simulink model "sampleModel223"  (R2021b)
settings: Solver=VariableStepAuto  StartTime=0.0  StopTime=10.0  RelTol=1e-3
undefined symbols (not defined in the file or in its folder): DiscIntNeverNeededParam
libraries: simulink x6
settings Model: Creator=user  LastModifiedBy=user

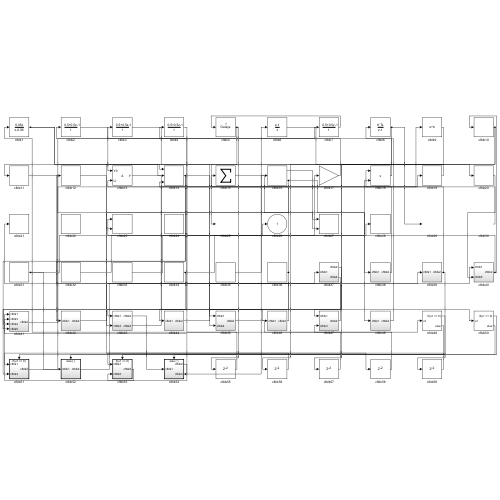
[thumbnail: Simulink's stored preview of the top-level diagram]
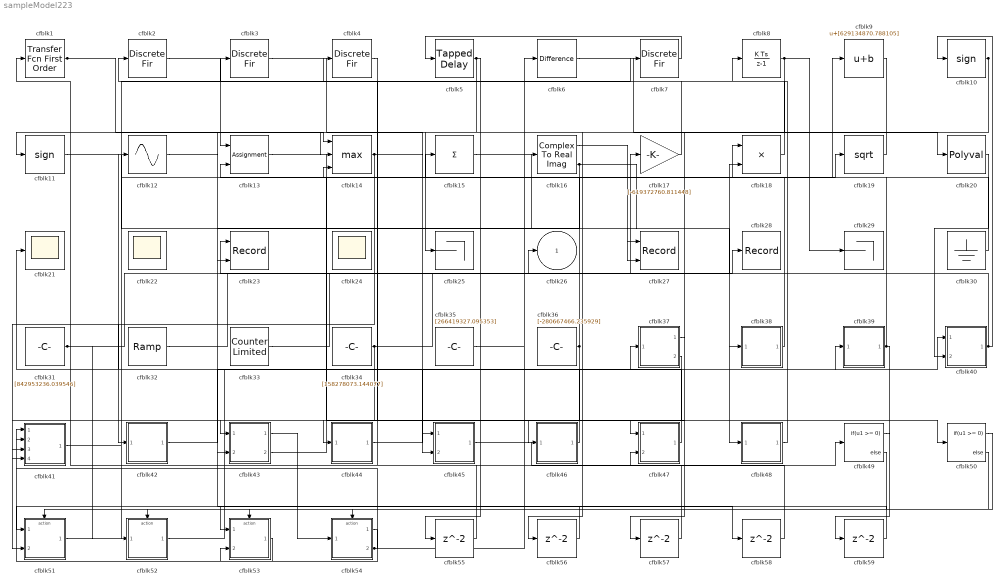
== system sampleModel223 ==
  cfblk1 : simulink/Discrete/Transfer Fcn First Order  PoleZ=0.95  ICPrevOutput=0.0  DoSatur=off
  cfblk10 : Signum
  cfblk11 : Signum
  cfblk12 : Sin  TimeSource=Use external signal  SampleTime=0
  cfblk13 : Assignment  DiagnosticForDimensions=Warning  IndexOptions=Index vector (dialog)  Indices=1  OutputSizes=1
  cfblk14 : MinMax  Function=max  Inputs=3
  cfblk15 : Sum  Inputs=+
  cfblk16 : ComplexToRealImag
  cfblk17 : Gain  Gain=[-619372760.811448]
  cfblk18 : Product
  cfblk19 : Sqrt  SaturateOnIntegerOverflow=on
  cfblk{2..4,7} (4 alike) : DiscreteFir  SampleTime=1
  cfblk20 : Polyval  Coefs=[ +2.081618890e-019, -1.441693666e-014, +4.719686976e-010, -8.536869453e-006, +1.621573104e-001, -8.087801117e+001 ]
  cfblk21 : Scope
  cfblk22 : Scope
      settings: Floating=on
  cfblk23 : Record  FileSettingsInternal="{\"entries\":[{\"content\":{\"excelSettings\":{\"content\":{},\"type\":\"Streamout.ExcelSettings\"}},\"type\":\"Streamout.FileSettingStorage\",\"uuid\":\"0ee5e5d3-5951-4c48-9d89-32d8b12ba518\"}],\"packageUris\":[\"http://schema.mathworks.com/mf0/streamout_blocks/R2020a\"],\"version\":\"1.0\"}"  Layout=[1 1]  SignalsInternal="{\"entries\":[{\"content\":{\"signals\":[{\"content\":{\"blockPath\":[\"sampleModel223/cfblk23\"],\"channel\":[],\"dimensions\":[1],\"domain\":\"sampleModel223/cfblk23\",\"lineColor\":\"#a2142f\",\"plots\":[1],\"port\":1,\"sid\":[\"\"],\"signalID\":8702,\"signalName\":\"cfblk40\"},\"type\":\"RecordBlkView.Signal\",\"uuid\":\"30bc6bd1-39a8-4b59-9cbd-2b18e3afbf50\"},{\"content\":{\"blockPath\":[\"sampleModel223/cfblk23\"],\"channel\":[],\"dimensions\":[1],\"domain\":\"sampleModel223/cfblk23\",\"lineColor\":\"#139fff\",\"plots\":[1],\"port\":2,\"sid\":[\"\"],\"signalID\":8706,\"signalName\":\"cfblk16:2\"},\"type\":\"RecordBlkView.Signal\",\"uuid\":\"da769030-c28c-44c7-86a2-4d1f259b478e\"}]},\"type\":\"RecordBlkView.InputSignals\",\"uuid\":\"dad23ff0-d1d3-46bd-a827-64e16703a200\"}],\"packageUris\":[\"http://schema.mathworks.com/mf0/streamout_blocks/R2020a\"],\"version\":\"1.0\"}"  VisualizationBindings="{\"xyplotplugin\":{\"info\":[{\"series\":[{\"bindingParametersList\":[{\"parameter\":\"X-Axis\",\"signalID\":8702,\"signalName\":\"cfblk40\"},{\"parameter\":\"Y-Axis\",\"signalID\":8706,\"signalName\":\"cfblk16:2\"}],\"seriesID\":59310}],\"subplotID\":1}]}}"  CompatibilityTag=XY
  cfblk24 : Scope
      settings: Floating=on
  cfblk25 : Terminator
  cfblk27 : Record  FileSettingsInternal="{\"entries\":[{\"content\":{\"excelSettings\":{\"content\":{},\"type\":\"Streamout.ExcelSettings\"}},\"type\":\"Streamout.FileSettingStorage\",\"uuid\":\"b9045ad8-1652-4b93-96d3-11a4ff897f15\"}],\"packageUris\":[\"http://schema.mathworks.com/mf0/streamout_blocks/R2020a\"],\"version\":\"1.0\"}"  Layout=[1 1]  SignalsInternal="{\"entries\":[{\"content\":{\"signals\":[{\"content\":{\"blockPath\":[\"sampleModel223/cfblk27\"],\"channel\":[],\"dimensions\":[1],\"domain\":\"sampleModel223/cfblk27\",\"lineColor\":\"#a2142f\",\"plots\":[1],\"port\":1,\"sid\":[\"\"],\"signalID\":8710,\"signalName\":\"cfblk16:1\"},\"type\":\"RecordBlkView.Signal\",\"uuid\":\"1ed41653-2a62-4b63-b81e-2f1a57827a1a\"},{\"content\":{\"blockPath\":[\"sampleModel223/cfblk27\"],\"channel\":[],\"dimensions\":[1],\"domain\":\"sampleModel223/cfblk27\",\"lineColor\":\"#139fff\",\"plots\":[1],\"port\":2,\"sid\":[\"\"],\"signalID\":8714,\"signalName\":\"cfblk11\"},\"type\":\"RecordBlkView.Signal\",\"uuid\":\"408a8370-a751-4b9d-9405-1cbd384d5eae\"}]},\"type\":\"RecordBlkView.InputSignals\",\"uuid\":\"9255ecad-2c20-41ba-b360-5dd1c328ef31\"}],\"packageUris\":[\"http://schema.mathworks.com/mf0/streamout_blocks/R2020a\"],\"version\":\"1.0\"}"  VisualizationBindings="{\"xyplotplugin\":{\"info\":[{\"series\":[{\"bindingParametersList\":[{\"parameter\":\"X-Axis\",\"signalID\":8710,\"signalName\":\"cfblk16:1\"},{\"parameter\":\"Y-Axis\",\"signalID\":8714,\"signalName\":\"cfblk11\"}],\"seriesID\":26914}],\"subplotID\":1}]}}"  CompatibilityTag=XY
  cfblk28 : Record  FileSettingsInternal="{\"entries\":[{\"content\":{\"excelSettings\":{\"content\":{},\"type\":\"Streamout.ExcelSettings\"}},\"type\":\"Streamout.FileSettingStorage\",\"uuid\":\"d52c9f09-3e23-41ac-822c-45c95d6e0353\"}],\"packageUris\":[\"http://schema.mathworks.com/mf0/streamout_blocks/R2020a\"],\"version\":\"1.0\"}"  SignalsInternal="{\"entries\":[{\"content\":{\"signals\":[{\"content\":{\"blockPath\":[\"sampleModel223/cfblk28\"],\"channel\":[],\"dimensions\":[1],\"domain\":\"sampleModel223/cfblk28\",\"lineColor\":\"#a2142f\",\"plots\":[1],\"port\":1,\"sid\":[\"\"],\"signalID\":8718,\"signalName\":\"cfblk33\"},\"type\":\"RecordBlkView.Signal\",\"uuid\":\"ab8a1c3b-5c01-4c72-8513-52e01dea01a3\"}]},\"type\":\"RecordBlkView.InputSignals\",\"uuid\":\"638a2006-718f-46db-b654-e0460e5be373\"}],\"packageUris\":[\"http://schema.mathworks.com/mf0/streamout_blocks/R2020a\"],\"version\":\"1.0\"}"  VisualizationBindings="{\"sparklinesplugin\":{\"info\":[{\"bindingParametersList\":[],\"subplotID\":1}]}}"
  cfblk29 : Terminator
  cfblk30 : Ground
  cfblk31 : Constant  Value=[842953236.039546]  SampleTime=1
  cfblk32 : simulink/Sources/Ramp  slope=[7363.193329]  start=[47.564520]  InitialOutput=[-118788.554960]
  cfblk33 : simulink/Sources/Counter Limited  uplimit=[327.000000]  tsamp=-1
  cfblk34 : Constant  Value=[158278073.144077]  SampleTime=1
  cfblk35 : Constant  Value=[266419327.095353]  SampleTime=1
  cfblk36 : Constant  Value=[-280667466.235929]  SampleTime=1
  cfblk37 : Subsystem
  cfblk38 : Subsystem
  cfblk39 : Subsystem
  cfblk40 : Subsystem
  cfblk41 : Subsystem
  cfblk42 : Subsystem
  cfblk43 : Subsystem
  cfblk44 : Subsystem
  cfblk45 : Subsystem
  cfblk46 : Subsystem
  cfblk47 : Subsystem
  cfblk48 : Subsystem
  cfblk49 : If  IfExpression=u1 >= 0  SampleTime=1
  cfblk5 : simulink/Discrete/Tapped Delay  vinit=0.0  samptime=-1  NumDelays=1  DelayOrder=Oldest  includeCurrent=off
  cfblk50 : If  IfExpression=u1 >= 0  SampleTime=1
  cfblk51 : Subsystem  TreatAsAtomicUnit=on
  cfblk52 : Subsystem  TreatAsAtomicUnit=on
  cfblk53 : Subsystem  TreatAsAtomicUnit=on
  cfblk54 : Subsystem  TreatAsAtomicUnit=on
  cfblk{55..59} (5 alike) : Delay  SampleTime=1
  cfblk6 : simulink/Discrete/Difference  ICPrevInput=0.0  OutMin=[]  OutMax=[]  OutDataTypeStr=Inherit: Inherit via back propagation  OutDataType=fixdt(1, 16)  OutScaling=2^-10  DoSatur=off
  cfblk8 : DiscreteIntegrator  ICPrevOutput=DiscIntNeverNeededParam  ICPrevScaledInput=DiscIntNeverNeededParam
  cfblk9 : Bias  Bias=[629134870.788105]
  cfblk26 : Outport
  wires:
  cfblk30/1 -> cfblk18/1
  cfblk34/1 -> cfblk17/1, cfblk41/3(cfblk4)
  cfblk19/1 -> cfblk11/1
  cfblk5/1 -> cfblk25/1, cfblk55/1
  cfblk52/1(cfblk2) -> cfblk39/1(cfblk1)
  cfblk18/1 -> cfblk2/1
  cfblk39/1(cfblk2) -> cfblk15/1, cfblk59/1
  cfblk53/1(cfblk2) -> cfblk41/1(cfblk1)
  cfblk9/1 -> cfblk47/1(cfblk1)
  cfblk13/1 -> cfblk50/1
  cfblk1/1 -> cfblk14/1, cfblk14/2
  cfblk7/1 -> cfblk5/1
  cfblk45/1(cfblk2) -> cfblk49/1
  cfblk3/1 -> cfblk45/1(cfblk1)
  cfblk33/1 -> cfblk28/1
  cfblk31/1 -> cfblk26/1, cfblk52/1(cfblk1)
  cfblk10/1 -> cfblk56/1, cfblk57/1
  cfblk32/1 -> cfblk18/2
  cfblk16/1 -> cfblk27/1
  cfblk37/1(cfblk2) -> cfblk43/1(cfblk1)
  cfblk2/1 -> cfblk13/1
  cfblk17/1 -> cfblk3/1
  cfblk38/1(cfblk2) -> cfblk13/2
  cfblk15/1 -> cfblk38/1(cfblk1)
  cfblk51/1(cfblk2) -> cfblk19/1
  cfblk6/1 -> cfblk20/1
  cfblk54/1(cfblk2) -> cfblk53/2(cfblk5)
  cfblk36/1 -> cfblk4/1, cfblk51/2(cfblk4)
  cfblk54/2(cfblk4) -> cfblk6/1, cfblk41/2(cfblk3)
  cfblk43/1(cfblk2) -> cfblk54/1(cfblk1)
  cfblk42/1(cfblk2) -> cfblk37/1(cfblk1)
  cfblk41/1(cfblk2) -> cfblk7/1
  cfblk16/2 -> cfblk48/1(cfblk1), cfblk23/2
  cfblk14/1 -> cfblk46/1(cfblk1), cfblk42/1(cfblk1), cfblk41/4(cfblk5)
  cfblk43/2(cfblk4) -> cfblk9/1
  cfblk11/1 -> cfblk27/2
  cfblk48/1(cfblk2) -> cfblk8/1
  cfblk44/1(cfblk2) -> cfblk40/1(cfblk1)
  cfblk40/1(cfblk2) -> cfblk10/1, cfblk23/1
  cfblk47/1(cfblk2) -> cfblk12/1
  cfblk46/1(cfblk2) -> cfblk21/1
  cfblk20/1 -> cfblk40/2(cfblk5)
  cfblk8/1 -> cfblk43/2(cfblk3), cfblk29/1
  cfblk37/2(cfblk4) -> cfblk45/2(cfblk4)
  cfblk35/1 -> cfblk16/1
  cfblk4/1 -> cfblk44/1(cfblk1)
  cfblk49/1 -> cfblk51/Action
  cfblk49/2 -> cfblk52/Action
  cfblk50/1 -> cfblk53/Action
  cfblk50/2 -> cfblk54/Action
  cfblk55/1 -> cfblk1/1
  cfblk56/1 -> cfblk53/1(cfblk1)
  cfblk57/1 -> cfblk14/3
  cfblk12/1 -> cfblk58/1
  cfblk58/1 -> cfblk47/2(cfblk3)
  cfblk59/1 -> cfblk51/1(cfblk1)

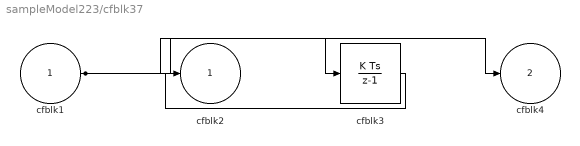
== system sampleModel223/cfblk37 ==
  cfblk1 : Inport
  cfblk3 : DiscreteIntegrator  ICPrevOutput=DiscIntNeverNeededParam  ICPrevScaledInput=DiscIntNeverNeededParam
  cfblk2 : Outport
  cfblk4 : Outport  Port=2
  wires:
  cfblk1/1 -> cfblk3/1, cfblk4/1
  cfblk3/1 -> cfblk2/1

== system sampleModel223/cfblk38 ==
  cfblk1 : Inport
  cfblk3 : simulink/Math Operations/MinMax Running Resettable  Function=min  vinit=0.0
  cfblk2 : Outport
  wires:
  cfblk1/1 -> cfblk2/1, cfblk3/1, cfblk3/2

== system sampleModel223/cfblk39 ==
  cfblk1 : Inport
  cfblk3 : Delay  ShowEnablePort=on  SampleTime=1
      settings: InputPortMap=u0,e6
  cfblk2 : Outport
  wires:
  cfblk1/1 -> cfblk3/1, cfblk3/2
  cfblk3/1 -> cfblk2/1

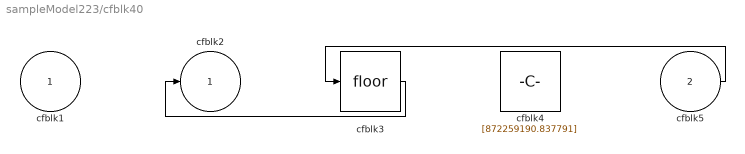
== system sampleModel223/cfblk40 ==
  cfblk1 : Inport
  cfblk5 : Inport  Port=2
  cfblk3 : Rounding
  cfblk4 : Constant  Value=[872259190.837791]  SampleTime=1
  cfblk2 : Outport
  wires:
  cfblk5/1 -> cfblk3/1
  cfblk3/1 -> cfblk2/1

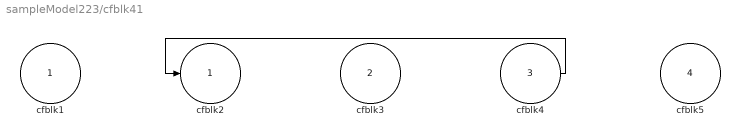
== system sampleModel223/cfblk41 ==
  cfblk1 : Inport
  cfblk3 : Inport  Port=2
  cfblk4 : Inport  Port=3
  cfblk5 : Inport  Port=4
  cfblk2 : Outport
  wires:
  cfblk4/1 -> cfblk2/1

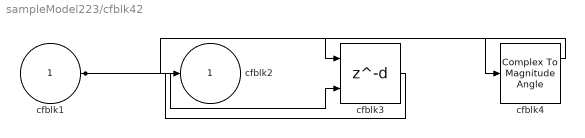
== system sampleModel223/cfblk42 ==
  cfblk1 : Inport
  cfblk3 : Delay  DelayLengthSource=Input port  SampleTime=1
      settings: InputPortMap=u0,p1
  cfblk4 : ComplexToMagnitudeAngle
  cfblk2 : Outport
  wires:
  cfblk4/1 -> cfblk3/1
  cfblk1/1 -> cfblk3/2, cfblk4/1
  cfblk3/1 -> cfblk2/1

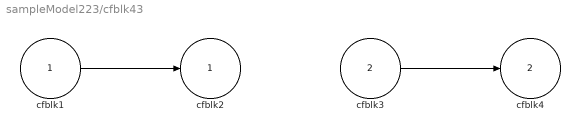
== system sampleModel223/cfblk43 ==
  cfblk1 : Inport
  cfblk3 : Inport  Port=2
  cfblk2 : Outport
  cfblk4 : Outport  Port=2
  wires:
  cfblk3/1 -> cfblk4/1
  cfblk1/1 -> cfblk2/1

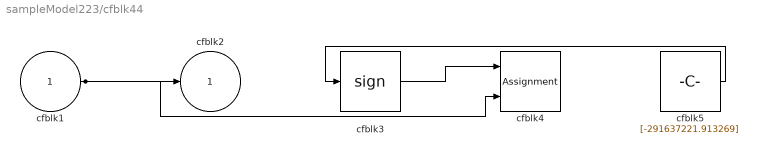
== system sampleModel223/cfblk44 ==
  cfblk1 : Inport
  cfblk3 : Signum
  cfblk4 : Assignment  DiagnosticForDimensions=Warning  IndexOptions=Index vector (dialog)  Indices=1  OutputSizes=1
  cfblk5 : Constant  Value=[-291637221.913269]  SampleTime=1
  cfblk2 : Outport
  wires:
  cfblk5/1 -> cfblk3/1
  cfblk3/1 -> cfblk4/1
  cfblk1/1 -> cfblk2/1, cfblk4/2

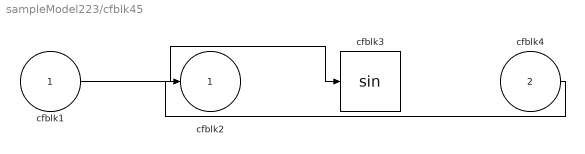
== system sampleModel223/cfblk45 ==
  cfblk1 : Inport
  cfblk4 : Inport  Port=2
  cfblk3 : Trigonometry
  cfblk2 : Outport
  wires:
  cfblk1/1 -> cfblk3/1
  cfblk4/1 -> cfblk2/1

== system sampleModel223/cfblk46 ==
  cfblk1 : Inport
  cfblk3 : UnaryMinus
  cfblk2 : Outport
  wires:
  cfblk3/1 -> cfblk2/1
  cfblk1/1 -> cfblk3/1

== system sampleModel223/cfblk47 ==
  cfblk1 : Inport
  cfblk3 : Inport  Port=2
  cfblk2 : Outport
  wires:
  cfblk1/1 -> cfblk2/1

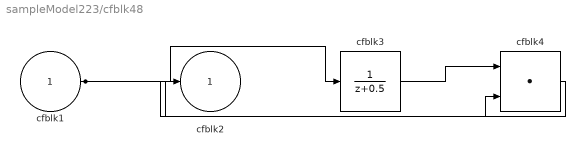
== system sampleModel223/cfblk48 ==
  cfblk1 : Inport
  cfblk3 : DiscreteTransferFcn  SampleTime=1
  cfblk4 : DotProduct  InputSameDT=on  OutDataTypeStr=Inherit: Inherit via internal rule
  cfblk2 : Outport
  wires:
  cfblk1/1 -> cfblk3/1, cfblk4/2
  cfblk3/1 -> cfblk4/1
  cfblk4/1 -> cfblk2/1

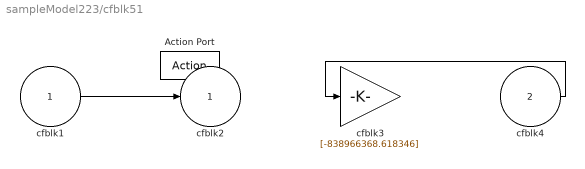
== system sampleModel223/cfblk51 ==
  cfblk1 : Inport
  cfblk4 : Inport  Port=2
  Action Port : ActionPort  ActionPortLabel=if(u1 >= 0)
  cfblk3 : Gain  Gain=[-838966368.618346]
  cfblk2 : Outport
  wires:
  cfblk1/1 -> cfblk2/1
  cfblk4/1 -> cfblk3/1

== system sampleModel223/cfblk52 ==
  cfblk1 : Inport
  Action Port : ActionPort  ActionPortLabel=else
  cfblk3 : DiscreteFilter
  cfblk2 : Outport
  wires:
  cfblk1/1 -> cfblk2/1, cfblk3/1

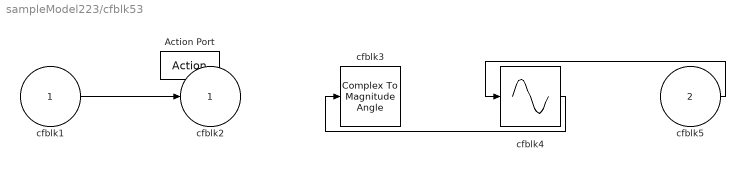
== system sampleModel223/cfblk53 ==
  cfblk1 : Inport
  cfblk5 : Inport  Port=2
  Action Port : ActionPort  ActionPortLabel=if(u1 >= 0)
  cfblk3 : ComplexToMagnitudeAngle
  cfblk4 : Sin  TimeSource=Use external signal  SampleTime=0
  cfblk2 : Outport
  wires:
  cfblk5/1 -> cfblk4/1
  cfblk1/1 -> cfblk2/1
  cfblk4/1 -> cfblk3/1

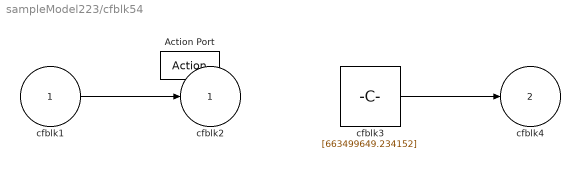
== system sampleModel223/cfblk54 ==
  cfblk1 : Inport
  Action Port : ActionPort  ActionPortLabel=else
  cfblk3 : Constant  Value=[663499649.234152]  SampleTime=1
  cfblk2 : Outport
  cfblk4 : Outport  Port=2
  wires:
  cfblk1/1 -> cfblk2/1
  cfblk3/1 -> cfblk4/1
